simulink model "UDPM_out"  (R2018b)
settings: Solver=FixedStepDiscrete  StartTime=0.0  StopTime=inf  FixedStep=0.01  RelTol=1e-3
undefined symbols (not defined in the file): selecting_parameters
libraries: etargetslib x1, dspnetwork x1
settings Model: Creator=Daniele Nava  LastModifiedBy=Daniele Nava

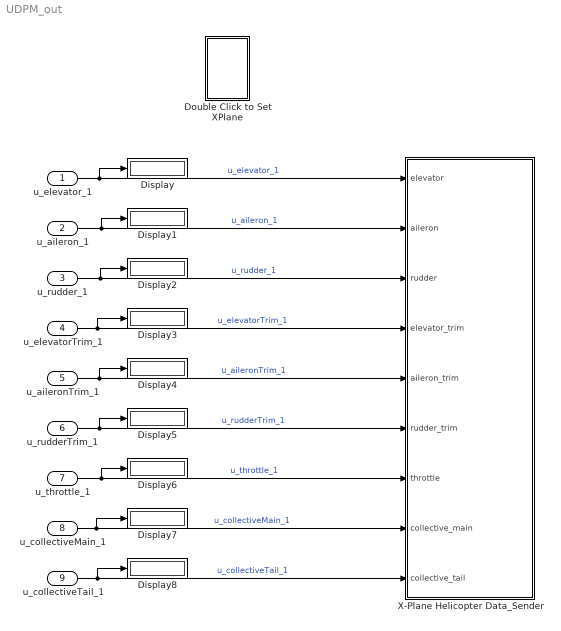
== system UDPM_out ==
  u_elevator_1 : Inport
  u_aileron_1 : Inport  Port=2
  u_rudder_1 : Inport  Port=3
  u_elevatorTrim_1 : Inport  Port=4
  u_aileronTrim_1 : Inport  Port=5
  u_rudderTrim_1 : Inport  Port=6
  u_throttle_1 : Inport  Port=7
  u_collectiveMain_1 : Inport  Port=8
  u_collectiveTail_1 : Inport  Port=9
  Display{,1..8} (9 alike) : Display
  Double Click to Set XPlane : Subsystem  LoadFcn=selecting_parameters()
      settings: OpenFcn=selecting_parameters()
  X-Plane Helicopter Data_Sender : Subsystem  mask{ip_address='127.0.0.1', port_number=49004, max_col_main=12, min_col_main=0, max_col_tail=5, min_col_tail=-5}
      mask prompts: ip_address "Local IP Address (default: '127.0.0.1' )"; port_number "Output Port Number (defaut: '49000')"; max_col_main "Max Angle For Collective Main"; min_col_main "Min Angle For Collective Main"; max_col_tail "Max Angle For Collective Tail"; min_col_tail "Min Angle For Collective Tail"
      mask help: This block is configured to send data to an helicopter aircraft on X-Plane Flight Simulator.
      mask Help: contact adrianobittar@gmail.com
  wires:
  u_elevator_1/1 -> Display/1, X-Plane Helicopter Data_Sender/1(elevator)  "u_elevator_1"
  u_aileron_1/1 -> Display1/1, X-Plane Helicopter Data_Sender/2(aileron)  "u_aileron_1"
  u_rudder_1/1 -> Display2/1, X-Plane Helicopter Data_Sender/3(rudder)  "u_rudder_1"
  u_elevatorTrim_1/1 -> Display3/1, X-Plane Helicopter Data_Sender/4(elevator_trim)  "u_elevatorTrim_1"
  u_aileronTrim_1/1 -> Display4/1, X-Plane Helicopter Data_Sender/5(aileron_trim)  "u_aileronTrim_1"
  u_rudderTrim_1/1 -> Display5/1, X-Plane Helicopter Data_Sender/6(rudder_trim)  "u_rudderTrim_1"
  u_throttle_1/1 -> Display6/1, X-Plane Helicopter Data_Sender/7(throttle)  "u_throttle_1"
  u_collectiveMain_1/1 -> X-Plane Helicopter Data_Sender/8(collective_main), Display7/1  "u_collectiveMain_1"
  u_collectiveTail_1/1 -> Display8/1, X-Plane Helicopter Data_Sender/9(collective_tail)  "u_collectiveTail_1"

== system UDPM_out/Double Click to Set XPlane ==

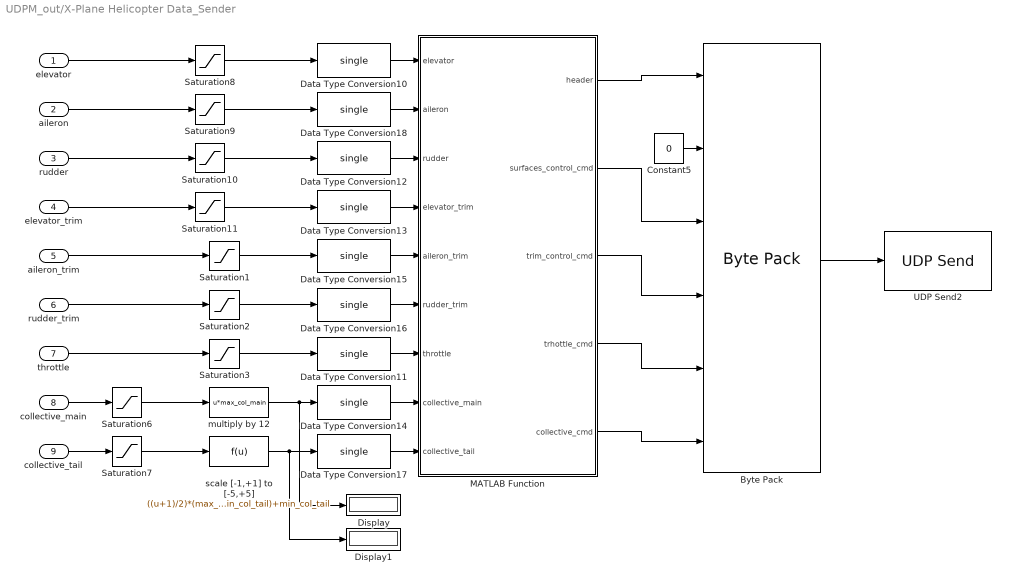
== system UDPM_out/X-Plane Helicopter Data_Sender ==
  elevator : Inport
  aileron : Inport  Port=2
  rudder : Inport  Port=3
  elevator_trim : Inport  Port=4
  aileron_trim : Inport  Port=5
  rudder_trim : Inport  Port=6
  throttle : Inport  Port=7
  collective_main : Inport  Port=8
  collective_tail : Inport  Port=9
  Byte Pack : etargetslib/Byte Pack  datatypes={'single','uint8','single','single','single','single'}  byteAlign=1
  Constant5 : Constant  Value=0  OutDataTypeStr=uint8
  Data Type Conversion{10..18} (9 alike) : DataTypeConversion  OutDataTypeStr=single  SaturateOnIntegerOverflow=on
  Display : Display
  Display1 : Display
  MATLAB Function : MATLAB Function  TreatAsAtomicUnit=on
  Saturation{1..3,6..11} (9 alike) : Saturate  UpperLimit=+1  LowerLimit=-1
  UDP Send2 : dspnetwork/UDP Send  remoteURL=ip_address  remotePort=port_number  localURL='255.255.255.255'  localPortSource=Automatically determine  localPort=-1  sampletime=-1  blockPlatform=HOST  separateLengthPort=0
      settings: SourceProductName=DSP System Toolbox  SourceProductBaseCode=DS
  multiply by 12 : Fcn  Expr=u*max_col_main
  scale [-1,+1] to [-5,+5] : Fcn  Expr=((u+1)/2)*(max_col_tail-min_col_tail)+min_col_tail
  wires:
  scale [-1,+1] to [-5,+5]/1 -> Display1/1, Data Type Conversion17/1
  throttle/1 -> Saturation3/1
  rudder_trim/1 -> Saturation2/1
  aileron_trim/1 -> Saturation1/1
  rudder/1 -> Saturation10/1
  multiply by 12/1 -> Display/1, Data Type Conversion14/1
  elevator/1 -> Saturation8/1
  Saturation2/1 -> Data Type Conversion16/1
  aileron/1 -> Saturation9/1
  Saturation1/1 -> Data Type Conversion15/1
  elevator_trim/1 -> Saturation11/1
  Saturation3/1 -> Data Type Conversion11/1
  collective_tail/1 -> Saturation7/1
  collective_main/1 -> Saturation6/1
  Saturation6/1 -> multiply by 12/1
  Saturation7/1 -> scale [-1,+1] to [-5,+5]/1
  Saturation9/1 -> Data Type Conversion18/1
  Saturation11/1 -> Data Type Conversion13/1
  Saturation10/1 -> Data Type Conversion12/1
  Data Type Conversion10/1 -> MATLAB Function/1(elevator)
  Data Type Conversion12/1 -> MATLAB Function/3(rudder)
  Data Type Conversion13/1 -> MATLAB Function/4(elevator_trim)
  Data Type Conversion15/1 -> MATLAB Function/5(aileron_trim)
  Data Type Conversion16/1 -> MATLAB Function/6(rudder_trim)
  Data Type Conversion11/1 -> MATLAB Function/7(throttle)
  Data Type Conversion14/1 -> MATLAB Function/8(collective_main)
  Data Type Conversion17/1 -> MATLAB Function/9(collective_tail)
  Byte Pack/1 -> UDP Send2/1
  MATLAB Function/1(header) -> Byte Pack/1
  MATLAB Function/2(surfaces_control_cmd) -> Byte Pack/3
  MATLAB Function/3(trim_control_cmd) -> Byte Pack/4
  MATLAB Function/4(trhottle_cmd) -> Byte Pack/5
  MATLAB Function/5(collective_cmd) -> Byte Pack/6
  Constant5/1 -> Byte Pack/2
  Data Type Conversion18/1 -> MATLAB Function/2(aileron)
  Saturation8/1 -> Data Type Conversion10/1

== matlab function UDPM_out/X-Plane Helicopter Data_Sender/MATLAB Function ==
  data: elevator input single size=1; aileron input; rudder input; elevator_trim input; aileron_trim input; rudder_trim input; throttle input; collective_main input; collective_tail input; header output single size=1; surfaces_control_cmd output single size=[1 18]; trim_control_cmd output single size=[1 18]; trhottle_cmd output single size=[1 9]; collective_cmd output single size=[1 9]
function [header, surfaces_control_cmd,trim_control_cmd,trhottle_cmd,collective_cmd]  = fcn(elevator, aileron, rudder, elevator_trim, aileron_trim, rudder_trim, throttle, collective_main, collective_tail)
% This block supports the Embedded MATLAB subset.
% See the help menu for details. 

header = typecast(uint8([uint8(68) uint8(65) uint8(84) uint8(65)]), 'single');




No_Comand = single(-999);

Surface_header = typecast(uint8([uint8(8) uint8(0) uint8(0) uint8(0)]), 'single');

surfaces_control_cmd = [Surface_header elevator aileron rudder No_Comand No_Comand No_Comand No_Comand No_Comand Surface_header No_Comand No_Comand No_Comand No_Comand No_Comand No_Comand No_Comand No_Comand];

Trim_header = typecast(uint8([uint8(13) uint8(0) uint8(0) uint8(0)]), 'single');


trim_control_cmd = [ Trim_header elevator_trim aileron_trim rudder_trim No_Comand No_Comand No_Comand No_Comand No_Comand Trim_header No_Comand No_Comand No_Comand No_Comand No_Comand No_Comand No_Comand No_Comand];

Throttle_header = typecast(uint8([uint8(25) uint8(0) uint8(0) uint8(0)]), 'single');
trhottle_cmd = [Throttle_header throttle No_Comand No_Comand No_Comand No_Comand No_Comand No_Comand No_Comand];

Collective_header = typecast(uint8([uint8(39) uint8(0) uint8(0) uint8(0)]), 'single');

collective_cmd = [ Collective_header collective_main collective_tail No_Comand No_Comand No_Comand No_Comand No_Comand No_Comand];
%data_out = [surfaces_control_cmd trim_control_cmd trhottle_cmd collective_cmd];


% Actuadors_Out[0] = 68;
% Actuadors_Out[1] = 65;
% Actuadors_Out[2] = 84;
% Actuadors_Out[3] = 65;
% Actuadors_Out[4] = 48;//26;
% aileron = data_in(3,1);
% rudder= data_in(4,1);
% 
% 
% elevator_trim= data_in(2,2);
% aileron_trim= data_in(3,2);
% rudder_trim= data_in(4,2);
% 
% q= data_in(2,3);
% p= data_in(3,3);
% r= data_in(4,3);
% 
% pitch= data_in(2,4);
% roll= data_in(3,4);
% heading_true= data_in(4,4);
% 
% Px= data_in(2,5);
% Py= data_in(3,5);
% Pz= data_in(4,5);
% Vx= data_in(5,5);
% Vy= data_in(6,5);
% Vz= data_in(7,5);
% 
% collective_main= data_in(2,6);
% collective_tail= data_in(3,6);
